simulink subsystem "SLembaInterface"  (R2024a)
settings: Solver=VariableStepAuto  StartTime=0.0  StopTime=10.0  RelTol=1e-3
undefined symbols (not defined in the file or in its folder): HS, IO291, RollOffset
libraries: speedgoatlib_IO691 x3, aru_toolbox x2, Heather_changed x2, eeGeneralControl x2, speedgoatlib_IO291 x1
settings Model: Creator=user  LastModifiedBy=user

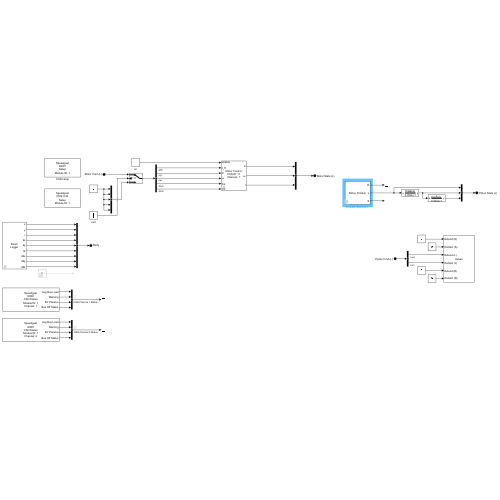
[thumbnail: Simulink's stored preview of the top-level diagram]
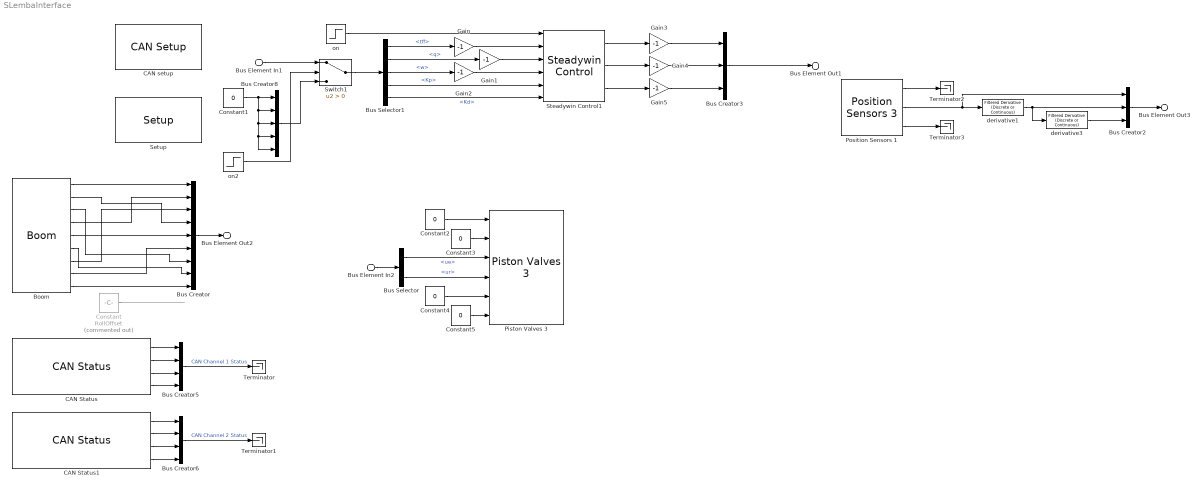
== system SLembaInterface ==
  Bus Element In1 : Inport  PortName=Motor Cmd (L)
  Bus Element In2 : Inport  Port=2  PortName=Piston Cmd (L)
  Boom : aru_toolbox/Boom  ts=0.001
      link override Serial Read HW FIFO: pciSlot=-1  board=IO393-50k
      link override Serial Setup: pciSlot=-1  board=IO393-50k
      settings: SourceProductName=ARU Toolbox
  Bus Creator : BusCreator  Inputs=9  OutDataTypeStr=Bus: BodyState  NonVirtualBus=on
      settings: InheritFromInputs=off
  Bus Creator2 : BusCreator  Inputs=3  OutDataTypeStr=Bus: PistonState  NonVirtualBus=on
      settings: InheritFromInputs=off
  Bus Creator3 : BusCreator  Inputs=3  OutDataTypeStr=Bus: MotorState  NonVirtualBus=on
      settings: InheritFromInputs=off
  Bus Creator5 : BusCreator  Inputs=4  OutDataTypeStr=Bus: CAN  NonVirtualBus=on
      settings: InheritFromInputs=off
  Bus Creator6 : BusCreator  Inputs=4  OutDataTypeStr=Bus: CAN  NonVirtualBus=on
      settings: InheritFromInputs=off
  Bus Creator8 : BusCreator  Inputs=5  OutDataTypeStr=Bus: MotorCmd  NonVirtualBus=on
      settings: InheritFromInputs=off
  Bus Selector : BusSelector  OutputSignals=ue,ur
  Bus Selector1 : BusSelector  OutputSignals=tff,q,w,Kp,Kd
  CAN Status : speedgoatlib_IO691/Legacy/CAN Status  moduleId=1  sampleTime=0.001  channel=1  busRecovery=Auto  arrayOutput=off  controllerCpuLoad=off  controllerLiveCount=off  initModeAct=off  avgBusLoad=on  receiving=off  RxQueueEmpty=off  dataOverrunRcv=off  rxBufferLevel=off  txPending=off  dataOverrunTx=off  txBufferLevel=off  errWarnLimit=on  errPassLimit=on  errBusOff=on  busRecoveryCounter=off  busCouplingErr=off  transceiverErr=off  opMode=off  brp=off  timeSegment1=off  timeSegment2=off  synchronisationJumpWidth=off  dataTSEG1=off  dataTSEG2=off  dataSJW=off  moduleType=691  qtyStatBlk=1  ptIdx=0  isFDMod=0
      settings: SourceProductName=IO691
  CAN Status1 : speedgoatlib_IO691/Legacy/CAN Status  moduleId=1  sampleTime=0.001  channel=2  busRecovery=Auto  arrayOutput=off  controllerCpuLoad=off  controllerLiveCount=off  initModeAct=off  avgBusLoad=on  receiving=off  RxQueueEmpty=off  dataOverrunRcv=off  rxBufferLevel=off  txPending=off  dataOverrunTx=off  txBufferLevel=off  errWarnLimit=on  errPassLimit=on  errBusOff=on  busRecoveryCounter=off  busCouplingErr=off  transceiverErr=off  opMode=off  brp=off  timeSegment1=off  timeSegment2=off  synchronisationJumpWidth=off  dataTSEG1=off  dataTSEG2=off  dataSJW=off  moduleType=691  qtyStatBlk=1  ptIdx=0  isFDMod=0
      settings: SourceProductName=IO691
  CAN setup : speedgoatlib_IO691/Legacy/CAN Setup   moduletype=IO691  id=1  pciSlot=-1  chn1=CAN (HS)  chn2=CAN (HS)  chn3=Disabled  chn4=Disabled  initStruct=[]  termStruct=[struct('Channel',1,'Protocol','CAN','BRS',0,'Type','Standard','Identifier',1,'Data',[255, 255, 255, 255, 255, 255, 255, 253],'Pause',0.001), struct('Channel',2,'Protocol','CAN','BRS',0,'Type','Standard','Identifier',2,'Data',[255, 255, 255, 255, 255, 255, 255, 253],'Pause',0.001)]  ArbitrationbdrChn1=1.0 MBaud  ArbitrationManbdrChn1=[2,8,31,8]  FdbdrChn1=1.0 MBaud  FdManbdrChn1=[2,8,31,8]  ArbitrationbdrChn2=1.0 MBaud  ArbitrationManbdrChn2=[2,8,31,8]  FdbdrChn2=1.0 MBaud  FdManbdrChn2=[2,8,31,8]  ArbitrationbdrChn3=1.0 MBaud  ArbitrationManbdrChn3=[2,8,31,8]  FdbdrChn3=5.0 MBaud  FdManbdrChn3=[2,2,5,2]  ArbitrationbdrChn4=1.0 MBaud  ArbitrationManbdrChn4=[2,8,31,8]  FdbdrChn4=5.0 MBaud  FdManbdrChn4=[2,2,5,2]  moduleInitValues=[691 1 -1 -1]
      settings: SourceProductName=IO691
  Constant : Constant  Commented=on  Value=RollOffset
  Constant1 : Constant  Value=0  SampleTime=0
  Constant{2..5} (4 alike) : Constant  Value=0
  Gain{,1..5} (6 alike) : Gain  Gain=-1
  Piston Valves 3 : Heather_changed/Piston Valves 3  SystemSampleTime=-1  VariantActivationTime=update diagram  AllowFlexibleInterface=on  Latency=0  AutoFrameSizeCalculation=off
      link override "solenoids ": parInternalModuleId=1
  Position Sensors 1 : Heather_changed/Position Sensors 3  stroke1=0.07  min_r=800  max_r=3695  stroke2=0.07  min_l=800  max_l=3695  stroke3=0.2  min_s=741  max_s=3392
  "Setup " : speedgoatlib_IO291/Setup   parInternalModuleId=1  parPciSlot=-1  parModuleId=1  parModuleType=IO291-HS  parTtlDoChannels=[]  parTtlDoInitValues=1  parTtlDoReset=1  parTtlDiChannels=[1 2 3 4 5]  parIsolDiChannels=[]  parFetDoChannels=[1 2 3 4 5 6]  parFetDoInitValues=0  parFetDoReset=1
      settings: SourceProductName=IO291
  Steadywin Control1 : aru_toolbox/Steadywin Control  id=10  channel=2  offset=0
      settings: SourceProductName=ARU Toolbox
  Switch1 : Switch  Criteria=u2 > Threshold  SaturateOnIntegerOverflow=off  InputSameDT=off
  Terminator{,1..3} (4 alike) : Terminator
  derivative1 : eeGeneralControl/Filtered Derivative (Discrete or Continuous)  K=1  T=0.002  B=inf  A=-inf  minRatio=2  init_option=Inherited from block input  x0=0  Ts=0.001
  derivative3 : eeGeneralControl/Filtered Derivative (Discrete or Continuous)  K=1  T=0.002  B=inf  A=-inf  minRatio=2  init_option=Inherited from block input  x0=0  Ts=0.001
  on : Step  SampleTime=0
  on2 : Step  Time=2.2  SampleTime=0
  Bus Element Out1 : Outport  PortName=Motor State (L)
  Bus Element Out3 : Outport  Port=2  PortName=Piston State (L)
  Bus Element Out2 : Outport  Port=3  PortName=Body
  wires:
  Steadywin Control1/1 -> Gain3/1
  Bus Selector/2 -> Piston Valves 3/4  "<ur>"
  Boom/3 -> Bus Creator/7
  Steadywin Control1/3 -> Gain5/1
  Bus Creator6/1 -> Terminator1/1  "CAN Channel 2 Status"
  CAN Status1/3 -> Bus Creator6/3
  Position Sensors 1/3 -> Terminator3/1
  Bus Element In2/1 -> Bus Selector/1
  Bus Creator2/1 -> Bus Element Out3/1
  Boom/1 -> Bus Creator/1
  Steadywin Control1/2 -> Gain4/1
  CAN Status/2 -> Bus Creator5/2
  Constant/1 -> ?
  Bus Selector1/3 -> Gain2/1  "<w>"
  on/1 -> Steadywin Control1/1
  Boom/4 -> Bus Creator/2
  Boom/2 -> Bus Creator/4
  derivative3/1 -> Bus Creator2/3
  Boom/9 -> Bus Creator/9
  CAN Status1/2 -> Bus Creator6/2
  Bus Selector1/5 -> Steadywin Control1/6  "<Kd>"
  derivative1/1 -> Bus Creator2/2, derivative3/1
  CAN Status/1 -> Bus Creator5/1
  Boom/6 -> Bus Creator/8
  CAN Status/4 -> Bus Creator5/4
  Bus Selector/1 -> Piston Valves 3/3  "<ue>"
  CAN Status1/1 -> Bus Creator6/1
  Bus Creator5/1 -> Terminator/1  "CAN Channel 1 Status"
  Bus Element In1/1 -> Switch1/1
  Bus Selector1/4 -> Steadywin Control1/5  "<Kp>"
  CAN Status1/4 -> Bus Creator6/4
  Boom/8 -> Bus Creator/6
  Bus Selector1/2 -> Gain1/1  "<q>"
  Bus Selector1/1 -> Gain/1  "<tff>"
  Bus Creator/1 -> Bus Element Out2/1
  Boom/5 -> Bus Creator/5
  Position Sensors 1/2 -> Bus Creator2/1, derivative1/1
  CAN Status/3 -> Bus Creator5/3
  Constant1/1 -> Bus Creator8/1, Bus Creator8/2, Bus Creator8/3, Bus Creator8/4, Bus Creator8/5
  Bus Creator8/1 -> Switch1/3
  on2/1 -> Switch1/2
  Switch1/1 -> Bus Selector1/1
  Constant2/1 -> Piston Valves 3/1
  Constant3/1 -> Piston Valves 3/2
  Constant4/1 -> Piston Valves 3/5
  Constant5/1 -> Piston Valves 3/6
  Position Sensors 1/1 -> Terminator2/1
  Gain/1 -> Steadywin Control1/2
  Gain1/1 -> Steadywin Control1/3
  Gain2/1 -> Steadywin Control1/4
  Gain3/1 -> Bus Creator3/1
  Gain4/1 -> Bus Creator3/2
  Gain5/1 -> Bus Creator3/3
  Bus Creator3/1 -> Bus Element Out1/1
  Boom/7 -> Bus Creator/3
